simulink model "PID_voltage_controller_effective_stiffness"  (R2020b)
settings: Solver=VariableStepAuto  StartTime=0.0  StopTime=5  RelTol=1e-4
values from neighbouring files (symbols this model uses):
  beta = 2e-4    (= 0.0002)    [nonlinear_msd_run.m]
  c = 0.001    [nonlinear_msd_run.m]
  k = 100    [nonlinear_msd_run.m]
  m = .01    (= 0.01)    [nonlinear_msd_run.m]
undefined symbols (not defined in the file or in its folder): b
libraries: pid_lib x2, cstblocks x1
settings Model: Creator=Daniel  LastModifiedBy=Daniel
settings SolverCC: MaxConsecutiveMinStep=100

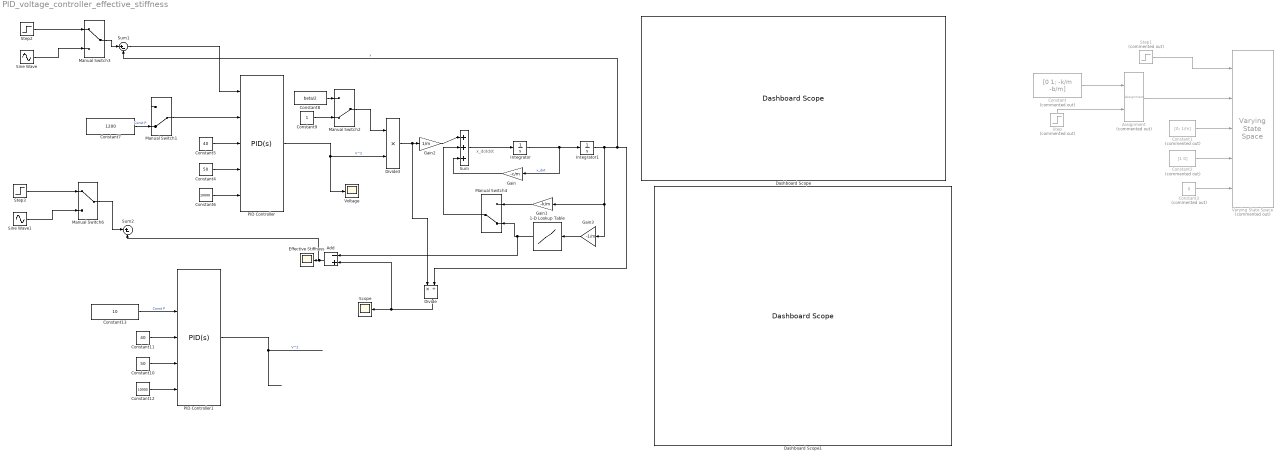
== system PID_voltage_controller_effective_stiffness ==
  note: x_dotdot
  1-D Lookup Table : Lookup_n-D  NumberOfTableDimensions=1  BreakpointsForDimension1=[-0.5:0.01:0.5]  Table=10*sin(2*[-0.5:0.01:0.5])+10  InternalRulePriority=Speed  RndMeth=Simplest  InputSameDT=on
  Add : Sum  Inputs=-+
  Assignment : Assignment  Commented=on  NumberOfDimensions=2  DiagnosticForDimensions=Warning  IndexOptions=Index vector (dialog),Index vector (dialog)  Indices=2,1  OutputSizes=1,1
  Constant : Constant  Commented=on  Value=[0 1; -k/m -b/m]
  Constant1 : Constant  Commented=on  Value=[0; 1/m]
  Constant10 : Constant  Value=50
  Constant11 : Constant  Value=40
  Constant12 : Constant  Value=10000
  Constant13 : Constant  Value=10
  Constant2 : Constant  Commented=on  Value=[1 0]
  Constant3 : Constant  Commented=on  Value=0
  Constant4 : Constant  Value=50
  Constant5 : Constant  Value=40
  Constant6 : Constant  Value=10000
  Constant7 : Constant  Value=1200
  Constant8 : Constant  Value=beta/2
  Constant9 : Constant
  Dashboard Scope : DashboardScope
  Dashboard Scope1 : DashboardScope  Ymin=-1000  Ymax=1000
  Divide : Product  Inputs=*/
  Divide3 : Product  Inputs=**
  Effective Stiffness : Scope
  Gain : Gain  Gain=-c/m
  Gain1 : Gain  Gain=-k/m
  Gain2 : Gain  Gain=1/m
  Gain3 : Gain  Gain=-1/m
  Integrator : Integrator
  Integrator1 : Integrator
  Manual Switch1 : ManualSwitch  CurrentSetting=0
  Manual Switch2 : ManualSwitch  CurrentSetting=0
  Manual Switch3 : ManualSwitch
  Manual Switch4 : ManualSwitch  CurrentSetting=0
  Manual Switch6 : ManualSwitch
  PID Controller : pid_lib/PID Controller  Controller=PID  Form=Parallel  TimeDomain=Continuous-time  UseExternalTs=off  SampleTime=-1  IntegratorMethod=Forward Euler  FilterMethod=Forward Euler  ControllerParametersSource=external  P=31000  I=10000  D=0  UseFilter=on  N=100  TunerSelectOption=Transfer Function Based (PID Tuner App)  InitialConditionSource=internal  InitialConditionForIntegrator=0  InitialConditionForFilter=0  DifferentiatorICPrevScaledInput=0  ExternalReset=none  TrackingMode=off  Kt=1  LimitOutput=off  SatLimitsSource=internal  UpperSaturationLimit=100  LowerSaturationLimit=-100  LinearizeAsGain=on  AntiWindupMode=clamping  Kb=1  POutMin=[]  POutMax=[]  IOutMin=[]  IOutMax=[]  DOutMin=[]  DOutMax=[]  NOutMin=[]  NOutMax=[]  SumOutMin=[]  SumOutMax=[]  SaturationOutMin=[]  SaturationOutMax=[]  PParamMin=[]  PParamMax=[]  IParamMin=[]  IParamMax=[]  DParamMin=[]  DParamMax=[]  NParamMin=[]  NParamMax=[]  KbParamMin=[]  KbParamMax=[]  KtParamMin=[]  KtParamMax=[]  KbOutMin=[]  KbOutMax=[]  KtOutMin=[]  KtOutMax=[]  IntegratorOutMin=[]  IntegratorOutMax=[]  FilterOutMin=[]  FilterOutMax=[]  SumI1OutMin=[]  SumI1OutMax=[]  SumI2OutMin=[]  SumI2OutMax=[]  SumI3OutMin=[]  SumI3OutMax=[]  SumI4OutMin=[]  SumI4OutMax=[]  SumDOutMin=[]  SumDOutMax=[]  DifferentiatorOutMin=[]  DifferentiatorOutMax=[]  FilterDiffOutCoefMin=[]  FilterDiffOutCoefMax=[]  ReciprocalOutMin=[]  ReciprocalOutMax=[]  SumDenOutMin=[]  SumDenOutMax=[]  SumNumOutMin=[]  SumNumOutMax=[]  DivideOutMin=[]  DivideOutMax=[]  UdiffTsProdOutMin=[]  UdiffTsProdOutMax=[]  NTsProdOutMin=[]  NTsProdOutMax=[]  UintegralTsProdOutMin=[]  UintegralTsProdOutMax=[]  UngainTsProdOutMin=[]  UngainTsProdOutMax=[]  IntegratorContinuousStateAttributes=''  IntegratorStateMustResolveToSignalObject=off  IntegratorRTWStateStorageClass=Auto  FilterContinuousStateAttributes=''  FilterStateMustResolveToSignalObject=off  FilterRTWStateStorageClass=Auto  ParallelPVariant=ExternalParameters  IdealPVariant=Disabled  IVariant=ExternalParameters  DVariant=ExternalParameters  IntegratorVariant=Continuous  SatVariant=Disabled  AWVariant=Passthrough  PCopyVariant=Disabled  TRVariant=Disabled  FdbkBlocksVariant=Forward  IdealPFdbkVariant=Disabled  SatFdbkVariant=Disabled  DerivativeFilterVariant=ContFilter  NVariant=ExternalParameters  NCopyVariant=Disabled  FilterICVariant=InternalICsFilter  IntegratorICVariant=InternalICs  ExternalResetVariant=Disabled  TRSumVariant=Passthrough  SumFdbkVariant=Disabled  SumVariant=Sum_PID  TsampFilterVariant=InternalTs  TsampNgainVariant=Passthrough  TsampIntegralVariant=Passthrough  ExternalSaturationOutDataTypeStr=Inherit: Same as second input
  PID Controller1 : pid_lib/PID Controller  Controller=PID  Form=Parallel  TimeDomain=Continuous-time  UseExternalTs=off  SampleTime=-1  IntegratorMethod=Forward Euler  FilterMethod=Forward Euler  ControllerParametersSource=external  P=31000  I=10000  D=0  UseFilter=on  N=100  TunerSelectOption=Transfer Function Based (PID Tuner App)  InitialConditionSource=internal  InitialConditionForIntegrator=0  InitialConditionForFilter=0  DifferentiatorICPrevScaledInput=0  ExternalReset=none  TrackingMode=off  Kt=1  LimitOutput=off  SatLimitsSource=internal  UpperSaturationLimit=100  LowerSaturationLimit=-100  LinearizeAsGain=on  AntiWindupMode=clamping  Kb=1  POutMin=[]  POutMax=[]  IOutMin=[]  IOutMax=[]  DOutMin=[]  DOutMax=[]  NOutMin=[]  NOutMax=[]  SumOutMin=[]  SumOutMax=[]  SaturationOutMin=[]  SaturationOutMax=[]  PParamMin=[]  PParamMax=[]  IParamMin=[]  IParamMax=[]  DParamMin=[]  DParamMax=[]  NParamMin=[]  NParamMax=[]  KbParamMin=[]  KbParamMax=[]  KtParamMin=[]  KtParamMax=[]  KbOutMin=[]  KbOutMax=[]  KtOutMin=[]  KtOutMax=[]  IntegratorOutMin=[]  IntegratorOutMax=[]  FilterOutMin=[]  FilterOutMax=[]  SumI1OutMin=[]  SumI1OutMax=[]  SumI2OutMin=[]  SumI2OutMax=[]  SumI3OutMin=[]  SumI3OutMax=[]  SumI4OutMin=[]  SumI4OutMax=[]  SumDOutMin=[]  SumDOutMax=[]  DifferentiatorOutMin=[]  DifferentiatorOutMax=[]  FilterDiffOutCoefMin=[]  FilterDiffOutCoefMax=[]  ReciprocalOutMin=[]  ReciprocalOutMax=[]  SumDenOutMin=[]  SumDenOutMax=[]  SumNumOutMin=[]  SumNumOutMax=[]  DivideOutMin=[]  DivideOutMax=[]  UdiffTsProdOutMin=[]  UdiffTsProdOutMax=[]  NTsProdOutMin=[]  NTsProdOutMax=[]  UintegralTsProdOutMin=[]  UintegralTsProdOutMax=[]  UngainTsProdOutMin=[]  UngainTsProdOutMax=[]  IntegratorContinuousStateAttributes=''  IntegratorStateMustResolveToSignalObject=off  IntegratorRTWStateStorageClass=Auto  FilterContinuousStateAttributes=''  FilterStateMustResolveToSignalObject=off  FilterRTWStateStorageClass=Auto  ParallelPVariant=ExternalParameters  IdealPVariant=Disabled  IVariant=ExternalParameters  DVariant=ExternalParameters  IntegratorVariant=Continuous  SatVariant=Disabled  AWVariant=Passthrough  PCopyVariant=Disabled  TRVariant=Disabled  FdbkBlocksVariant=Forward  IdealPFdbkVariant=Disabled  SatFdbkVariant=Disabled  DerivativeFilterVariant=ContFilter  NVariant=ExternalParameters  NCopyVariant=Disabled  FilterICVariant=InternalICsFilter  IntegratorICVariant=InternalICs  ExternalResetVariant=Disabled  TRSumVariant=Passthrough  SumFdbkVariant=Disabled  SumVariant=Sum_PID  TsampFilterVariant=InternalTs  TsampNgainVariant=Passthrough  TsampIntegralVariant=Passthrough  ExternalSaturationOutDataTypeStr=Inherit: Same as second input
  Scope : Scope
  Sine Wave : Sin  Amplitude=.1  Frequency=50  SampleTime=0
  Sine Wave1 : Sin  Amplitude=.1  Frequency=50  SampleTime=0
  Step : Step  Commented=on  SampleTime=0
  Step1 : Step  Commented=on  SampleTime=0
  Step2 : Step  After=.1  SampleTime=0
  Step3 : Step  After=1200  SampleTime=0
  Sum : Sum  Inputs=|+++
  Sum1 : Sum  Inputs=|+-
  Sum2 : Sum  Inputs=|+-
  Varying State Space : cstblocks/Linear Parameter Varying/Varying State Space  Commented=on  x0=[0; 0]  xNames=''  OutputX=on  OutputDX=on
  Voltage : Scope
  wires:
  Constant/1 -> Assignment/1
  Step/1 -> Assignment/2
  Assignment/1 -> Varying State Space/2
  Constant1/1 -> Varying State Space/3
  Constant2/1 -> Varying State Space/4
  Constant3/1 -> Varying State Space/5
  Step1/1 -> Varying State Space/1
  Gain2/1 -> Sum/1
  Integrator1/1 -> Divide/2, Sum1/2, Gain3/1, Gain1/1  "x"
  Sum/1 -> Integrator/1
  Gain/1 -> Sum/3
  Integrator/1 -> Gain/1, Integrator1/1  "x_dot"
  Constant5/1 -> PID Controller/3
  Constant6/1 -> PID Controller/5
  Constant4/1 -> PID Controller/4
  Constant7/1 -> Manual Switch1/2  "Const P"
  Manual Switch1/1 -> PID Controller/2
  Sum1/1 -> PID Controller/1
  Divide3/1 -> Divide/1, Gain2/1
  PID Controller/1 -> Voltage/1, Divide3/2  "V^2"
  Manual Switch2/1 -> Divide3/1
  Constant8/1 -> Manual Switch2/1
  Constant9/1 -> Manual Switch2/2
  Step2/1 -> Manual Switch3/1
  Sine Wave/1 -> Manual Switch3/2
  Manual Switch3/1 -> Sum1/1
  Gain1/1 -> Manual Switch4/1
  Manual Switch4/1 -> Sum/2
  1-D Lookup Table/1 -> Add/1, Manual Switch4/2
  Gain3/1 -> 1-D Lookup Table/1
  Divide/1 -> Add/2, Scope/1
  Add/1 -> Sum2/2, Effective Stiffness/1
  Manual Switch6/1 -> Sum2/1
  Sine Wave1/1 -> Manual Switch6/2
  Step3/1 -> Manual Switch6/1
  Constant10/1 -> PID Controller1/4
  PID Controller1/1 -> ?  "V^2"
  Constant11/1 -> PID Controller1/3
  Constant13/1 -> PID Controller1/2  "Const P"
  Constant12/1 -> PID Controller1/5
